simulink model "infrarrojo"  (R2024a)
settings: Solver=VariableStepAuto  StartTime=0.0  StopTime=10.0  RelTol=1e-3
settings Model: Creator=Usuario_UMA  LastModifiedBy=julia
settings RTWCC: GPUComputeCapability=3.5

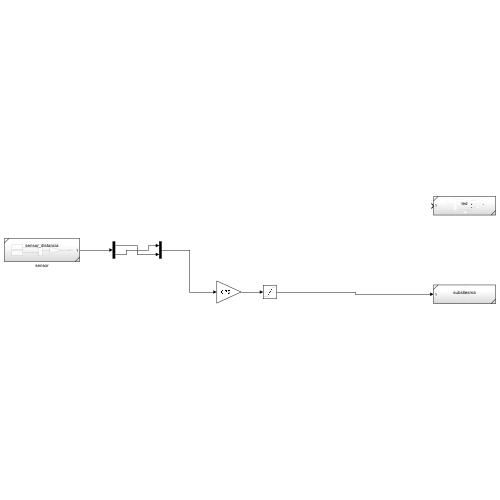
[thumbnail: Simulink's stored preview of the top-level diagram]
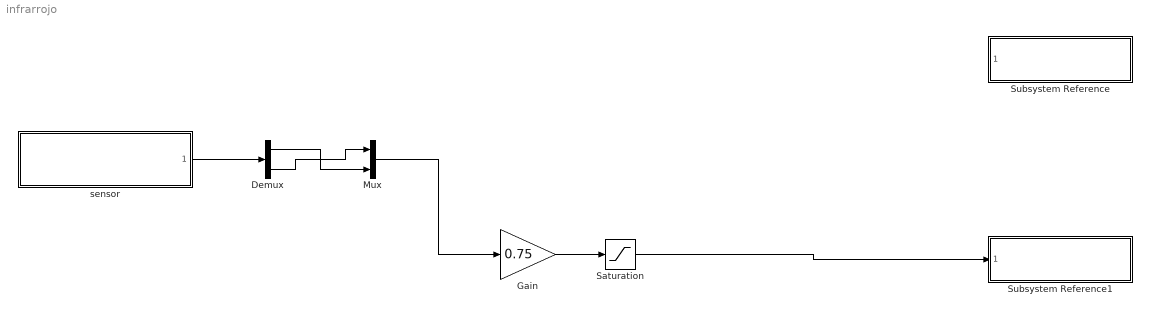
== system infrarrojo ==
  Demux : Demux  Outputs=2
  Gain : Gain  Gain=0.75
  Mux : Mux  Inputs=2
  Saturation : Saturate
  Subsystem Reference : Subsystem  ReferencedSubsystem=led
  Subsystem Reference1 : Subsystem  ReferencedSubsystem=subsitesma
  sensor : Subsystem  ReferencedSubsystem=sensor_distancia
  wires:
  sensor/1 -> Demux/1
  Demux/1 -> Mux/2
  Demux/2 -> Mux/1
  Mux/1 -> Gain/1
  Gain/1 -> Saturation/1
  Saturation/1 -> Subsystem Reference1/1
